simulink model "MON_sl"  (R2016a)
settings: Solver=FixedStepDiscrete  StartTime=0.0  StopTime=10.0  RelTol=1e-3
undefined symbols (not defined in the file): dt
Description:
  | BSCU Monitor Function Model
settings Model: ModelType=Feature  MBDTemplateVer=1.1  LastModifiedBy=jdbackes
settings DataIOCC: LimitDataPoints=on
settings DebuggingCC: AllowSymbolicDim=off
settings ModelReferenceCC: PropagateSignalLabelsOutOfModel=off
settings RTWCC: Description=Generic Real-Time Target
settings GRTTargetCC: GeneratePreprocessorConditionals=Use local settings
settings ConfigComp: DVMode=PropertyProving  DVTestSuiteOptimization=CombinedObjectives (Nonlinear Extended)  DVAssertions=EnableAll  DVProofAssumptions=EnableAll  DVDisplayReport=off

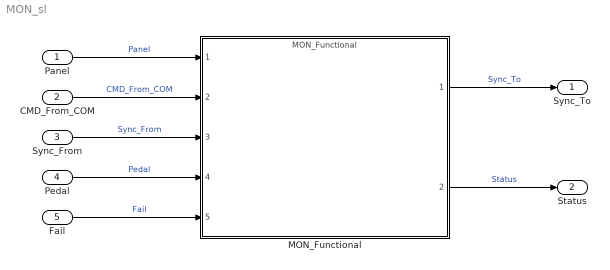
== system MON_sl ==
  Panel : Inport  OutDataTypeStr=Bus: PanelMsgImpl  SampleTime=dt  Interpolate=off  BusOutputAsStruct=on
  CMD_From_COM : Inport  Port=2  OutDataTypeStr=int32  SampleTime=dt  Interpolate=off
  Sync_From : Inport  Port=3  OutDataTypeStr=Bus: SyncMsgImpl  SampleTime=dt  Interpolate=off  BusOutputAsStruct=on
  Pedal : Inport  Port=4  OutDataTypeStr=int32  SampleTime=dt  Interpolate=off
  Fail : Inport  Port=5  OutDataTypeStr=boolean  SampleTime=dt  Interpolate=off
  MON_Functional : ModelReference  ModelNameDialog=MON_Functional.slx  SimulationMode=Normal  ModelReferenceVersion=1.2
  Sync_To : Outport  OutDataTypeStr=Bus: SyncMsgImpl  BusOutputAsStruct=on
  Status : Outport  Port=2  OutDataTypeStr=Bus: ChannelStatusImpl  BusOutputAsStruct=on
  wires:
  MON_Functional/1 -> Sync_To/1  "Sync_To"
  MON_Functional/2 -> Status/1  "Status"
  Panel/1 -> MON_Functional/1  "Panel"
  CMD_From_COM/1 -> MON_Functional/2  "CMD_From_COM"
  Sync_From/1 -> MON_Functional/3  "Sync_From"
  Pedal/1 -> MON_Functional/4  "Pedal"
  Fail/1 -> MON_Functional/5  "Fail"
